simulink model "pressure"  (Simulink 4.00)
settings: Solver=FixedStepDiscrete  StartTime=0.0  StopTime=5*length(u)  FixedStep=5  RelTol=1e-3
libraries: fuzblock x1

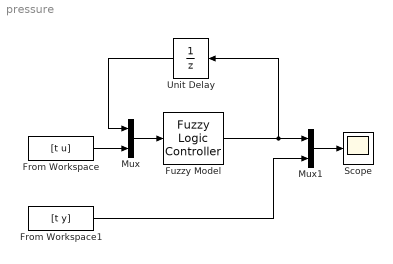
== system pressure ==
  From Workspace : FromWorkspace  VariableName=[t u]  SampleTime=5  OutputAfterFinalValue=Extrapolation
  From Workspace1 : FromWorkspace  VariableName=[t y]  SampleTime=5  OutputAfterFinalValue=Extrapolation
  Fuzzy Model : fuzblock/Fuzzy Logic  Controller  fis=FIS
  Mux : Mux  Inputs=2
  Mux1 : Mux  Inputs=2
  Scope : Scope
      settings: TimeRange=1500  YMin=1  YMax=2  SaveToWorkspace=off  SaveName=ScopeData  LimitDataPoints=on  MaxDataPoints=5000
  Unit Delay : UnitDelay  Orientation=left  X0=1  SampleTime=5
      settings: RTWStateStorageClass=Auto
  wires:
  Fuzzy Model/1 -> Unit Delay/1, Mux1/1
  Mux/1 -> Fuzzy Model/1
  Unit Delay/1 -> Mux/1
  From Workspace/1 -> Mux/2
  Mux1/1 -> Scope/1
  From Workspace1/1 -> Mux1/2
